simulink model "Funtivities"  (R2023b)
settings: Solver=VariableStepAuto  StartTime=0.0  StopTime=6  RelTol=1e-3
model workspace: external: MATLAB File D:\College\Senior 2\GP\Delta\Design\INSHALLAAHHHHH\SSCPE\Funtivities_DataFile3.m (data not in the file)
undefined symbols (not defined in the file or in its folder): smiData, X, Y, Z
libraries: sm_lib x231, nesl_utility x4
(part 5 of 5)

== system Funtivities/Delta Robot Model/Ta7t_1_RIGID/RodPlusTwoSpheres_2_RIGID ==
  ROd_1_RIGID : Subsystem
  ReferenceFrame : sm_lib/Frames and Transforms/Reference Frame
  Sphere_1_RIGID : Subsystem
  Sphere_2_RIGID : Subsystem
  Transform : sm_lib/Frames and Transforms/Rigid Transform  TranslationMethod=Cartesian  TranslationStandardOffset=0  TranslationStandardOffsetUnits=m  TranslationStandardAxis=+Z  TranslationCartesianOffset=smiData.RigidTransform(59).translation  TranslationCartesianOffsetUnits=mm  TranslationROffset=0  TranslationROffsetUnits=m  TranslationZOffset=0  TranslationZOffsetUnits=m  TranslationThetaOffset=0  TranslationThetaOffsetUnits=deg  RotationMethod=ArbitraryAxis  RotationAngleUnits=rad  RotationStandardAxis=+Z  RotationAngle=smiData.RigidTransform(59).angle  RotationArbitraryAxis=smiData.RigidTransform(59).axis  FollAlignAxisA=+X  BaseAlignAxisA=+Y  FollAlignAxisB=+Y  BaseAlignAxisB=+Z  RotationSequenceAxes=FollowerAxes  RotationSequence=XYX  RotationSequenceAngles=[0 0 0]  RotationSequenceAnglesUnits=deg  RotationMatrix=[1 0 0; 0 1 0; 0 0 1]  Quaternion=[1 0 0 0]
  Transform1 : sm_lib/Frames and Transforms/Rigid Transform  TranslationMethod=Cartesian  TranslationStandardOffset=0  TranslationStandardOffsetUnits=m  TranslationStandardAxis=+Z  TranslationCartesianOffset=smiData.RigidTransform(60).translation  TranslationCartesianOffsetUnits=mm  TranslationROffset=0  TranslationROffsetUnits=m  TranslationZOffset=0  TranslationZOffsetUnits=m  TranslationThetaOffset=0  TranslationThetaOffsetUnits=deg  RotationMethod=ArbitraryAxis  RotationAngleUnits=rad  RotationStandardAxis=+Z  RotationAngle=smiData.RigidTransform(60).angle  RotationArbitraryAxis=smiData.RigidTransform(60).axis  FollAlignAxisA=+X  BaseAlignAxisA=+Y  FollAlignAxisB=+Y  BaseAlignAxisB=+Z  RotationSequenceAxes=FollowerAxes  RotationSequence=XYX  RotationSequenceAngles=[0 0 0]  RotationSequenceAnglesUnits=deg  RotationMatrix=[1 0 0; 0 1 0; 0 0 1]  Quaternion=[1 0 0 0]
  Transform2 : sm_lib/Frames and Transforms/Rigid Transform  TranslationMethod=Cartesian  TranslationStandardOffset=0  TranslationStandardOffsetUnits=m  TranslationStandardAxis=+Z  TranslationCartesianOffset=smiData.RigidTransform(61).translation  TranslationCartesianOffsetUnits=mm  TranslationROffset=0  TranslationROffsetUnits=m  TranslationZOffset=0  TranslationZOffsetUnits=m  TranslationThetaOffset=0  TranslationThetaOffsetUnits=deg  RotationMethod=ArbitraryAxis  RotationAngleUnits=rad  RotationStandardAxis=+Z  RotationAngle=smiData.RigidTransform(61).angle  RotationArbitraryAxis=smiData.RigidTransform(61).axis  FollAlignAxisA=+X  BaseAlignAxisA=+Y  FollAlignAxisB=+Y  BaseAlignAxisB=+Z  RotationSequenceAxes=FollowerAxes  RotationSequence=XYX  RotationSequenceAngles=[0 0 0]  RotationSequenceAnglesUnits=deg  RotationMatrix=[1 0 0; 0 1 0; 0 0 1]  Quaternion=[1 0 0 0]
  Transform3 : sm_lib/Frames and Transforms/Rigid Transform  TranslationMethod=Cartesian  TranslationStandardOffset=0  TranslationStandardOffsetUnits=m  TranslationStandardAxis=+Z  TranslationCartesianOffset=smiData.RigidTransform(62).translation  TranslationCartesianOffsetUnits=mm  TranslationROffset=0  TranslationROffsetUnits=m  TranslationZOffset=0  TranslationZOffsetUnits=m  TranslationThetaOffset=0  TranslationThetaOffsetUnits=deg  RotationMethod=ArbitraryAxis  RotationAngleUnits=rad  RotationStandardAxis=+Z  RotationAngle=smiData.RigidTransform(62).angle  RotationArbitraryAxis=smiData.RigidTransform(62).axis  FollAlignAxisA=+X  BaseAlignAxisA=+Y  FollAlignAxisB=+Y  BaseAlignAxisB=+Z  RotationSequenceAxes=FollowerAxes  RotationSequence=XYX  RotationSequenceAngles=[0 0 0]  RotationSequenceAnglesUnits=deg  RotationMatrix=[1 0 0; 0 1 0; 0 0 1]  Quaternion=[1 0 0 0]
  F : PMIOPort  Side=Right
  connections:
  Sphere_1_RIGID/LConn1 -- Transform/RConn1
  Sphere_2_RIGID/LConn1 -- Transform1/RConn1
  ROd_1_RIGID/LConn1 -- Transform2/RConn1
  Transform/LConn1 -- ReferenceFrame/RConn1 -- Transform1/LConn1 -- Transform2/LConn1 -- Transform3/RConn1
  Transform3/LConn1 -- F/RConn1

== system Funtivities/Delta Robot Model/Ta7t_1_RIGID/RodPlusTwoSpheres_3_RIGID ==
  ROd_1_RIGID : Subsystem
  ReferenceFrame : sm_lib/Frames and Transforms/Reference Frame
  Sphere_1_RIGID : Subsystem
  Sphere_2_RIGID : Subsystem
  Transform : sm_lib/Frames and Transforms/Rigid Transform  TranslationMethod=Cartesian  TranslationStandardOffset=0  TranslationStandardOffsetUnits=m  TranslationStandardAxis=+Z  TranslationCartesianOffset=smiData.RigidTransform(63).translation  TranslationCartesianOffsetUnits=mm  TranslationROffset=0  TranslationROffsetUnits=m  TranslationZOffset=0  TranslationZOffsetUnits=m  TranslationThetaOffset=0  TranslationThetaOffsetUnits=deg  RotationMethod=ArbitraryAxis  RotationAngleUnits=rad  RotationStandardAxis=+Z  RotationAngle=smiData.RigidTransform(63).angle  RotationArbitraryAxis=smiData.RigidTransform(63).axis  FollAlignAxisA=+X  BaseAlignAxisA=+Y  FollAlignAxisB=+Y  BaseAlignAxisB=+Z  RotationSequenceAxes=FollowerAxes  RotationSequence=XYX  RotationSequenceAngles=[0 0 0]  RotationSequenceAnglesUnits=deg  RotationMatrix=[1 0 0; 0 1 0; 0 0 1]  Quaternion=[1 0 0 0]
  Transform1 : sm_lib/Frames and Transforms/Rigid Transform  TranslationMethod=Cartesian  TranslationStandardOffset=0  TranslationStandardOffsetUnits=m  TranslationStandardAxis=+Z  TranslationCartesianOffset=smiData.RigidTransform(64).translation  TranslationCartesianOffsetUnits=mm  TranslationROffset=0  TranslationROffsetUnits=m  TranslationZOffset=0  TranslationZOffsetUnits=m  TranslationThetaOffset=0  TranslationThetaOffsetUnits=deg  RotationMethod=ArbitraryAxis  RotationAngleUnits=rad  RotationStandardAxis=+Z  RotationAngle=smiData.RigidTransform(64).angle  RotationArbitraryAxis=smiData.RigidTransform(64).axis  FollAlignAxisA=+X  BaseAlignAxisA=+Y  FollAlignAxisB=+Y  BaseAlignAxisB=+Z  RotationSequenceAxes=FollowerAxes  RotationSequence=XYX  RotationSequenceAngles=[0 0 0]  RotationSequenceAnglesUnits=deg  RotationMatrix=[1 0 0; 0 1 0; 0 0 1]  Quaternion=[1 0 0 0]
  Transform2 : sm_lib/Frames and Transforms/Rigid Transform  TranslationMethod=Cartesian  TranslationStandardOffset=0  TranslationStandardOffsetUnits=m  TranslationStandardAxis=+Z  TranslationCartesianOffset=smiData.RigidTransform(65).translation  TranslationCartesianOffsetUnits=mm  TranslationROffset=0  TranslationROffsetUnits=m  TranslationZOffset=0  TranslationZOffsetUnits=m  TranslationThetaOffset=0  TranslationThetaOffsetUnits=deg  RotationMethod=ArbitraryAxis  RotationAngleUnits=rad  RotationStandardAxis=+Z  RotationAngle=smiData.RigidTransform(65).angle  RotationArbitraryAxis=smiData.RigidTransform(65).axis  FollAlignAxisA=+X  BaseAlignAxisA=+Y  FollAlignAxisB=+Y  BaseAlignAxisB=+Z  RotationSequenceAxes=FollowerAxes  RotationSequence=XYX  RotationSequenceAngles=[0 0 0]  RotationSequenceAnglesUnits=deg  RotationMatrix=[1 0 0; 0 1 0; 0 0 1]  Quaternion=[1 0 0 0]
  Transform3 : sm_lib/Frames and Transforms/Rigid Transform  TranslationMethod=Cartesian  TranslationStandardOffset=0  TranslationStandardOffsetUnits=m  TranslationStandardAxis=+Z  TranslationCartesianOffset=smiData.RigidTransform(66).translation  TranslationCartesianOffsetUnits=mm  TranslationROffset=0  TranslationROffsetUnits=m  TranslationZOffset=0  TranslationZOffsetUnits=m  TranslationThetaOffset=0  TranslationThetaOffsetUnits=deg  RotationMethod=ArbitraryAxis  RotationAngleUnits=rad  RotationStandardAxis=+Z  RotationAngle=smiData.RigidTransform(66).angle  RotationArbitraryAxis=smiData.RigidTransform(66).axis  FollAlignAxisA=+X  BaseAlignAxisA=+Y  FollAlignAxisB=+Y  BaseAlignAxisB=+Z  RotationSequenceAxes=FollowerAxes  RotationSequence=XYX  RotationSequenceAngles=[0 0 0]  RotationSequenceAnglesUnits=deg  RotationMatrix=[1 0 0; 0 1 0; 0 0 1]  Quaternion=[1 0 0 0]
  F : PMIOPort  Side=Right
  connections:
  Sphere_1_RIGID/LConn1 -- Transform/RConn1
  Sphere_2_RIGID/LConn1 -- Transform1/RConn1
  ROd_1_RIGID/LConn1 -- Transform2/RConn1
  Transform/LConn1 -- ReferenceFrame/RConn1 -- Transform1/LConn1 -- Transform2/LConn1 -- Transform3/RConn1
  Transform3/LConn1 -- F/RConn1

== system Funtivities/Delta Robot Model/Ta7t_1_RIGID/playe_1_RIGID ==
  ReferenceFrame : sm_lib/Frames and Transforms/Reference Frame
  Solid : sm_lib/Body Elements/File Solid  ExtGeomFileName=playe_Default_sldprt.STEP  UnitType=FromFile  ExtGeomFileUnits=m  StepReaderType=HEX  ExportConvexHullGeometry=off  InertiaType=Custom  Mass=smiData.Solid(9).mass  MassUnits=kg  CenterOfMass=smiData.Solid(9).CoM  CenterOfMassUnits=mm  MomentsOfInertia=smiData.Solid(9).MoI  MomentsOfInertiaUnits=kg*mm^2  ProductsOfInertia=smiData.Solid(9).PoI  ProductsOfInertiaUnits=kg*mm^2  BasedOnType=DensityFromFile  Density=1000  DensityUnits=kg/m^3  DoExposeReferenceFrame=on  SerializedFrames=<Frames/>  GraphicType=FromGeometry  MarkerShape=Sphere  MarkerSize=10  GraphicVisPropType=SimpleVisualProperties  GraphicDiffuseColor=smiData.Solid(9).color  GraphicSpecularColor=[0.5 0.5 0.5 1.0]  GraphicAmbientColor=[0.15 0.15 0.15 1.0]  GraphicEmissiveColor=[0.0 0.0 0.0 1.0]  GraphicShininess=75  GraphicOpacity=smiData.Solid(9).opacity
  F : PMIOPort  Side=Left
  connections:
  Solid/RConn1 -- ReferenceFrame/RConn1 -- F/RConn1

== system Funtivities/Delta Robot Model/Ta7t_1_RIGID/RodPlusTwoSpheres_1_RIGID/ROd_1_RIGID ==
  ReferenceFrame : sm_lib/Frames and Transforms/Reference Frame
  Solid : sm_lib/Body Elements/File Solid  ExtGeomFileName=ROd_Default_sldprt.STEP  UnitType=FromFile  ExtGeomFileUnits=m  StepReaderType=HEX  ExportConvexHullGeometry=off  InertiaType=Custom  Mass=smiData.Solid(8).mass  MassUnits=kg  CenterOfMass=smiData.Solid(8).CoM  CenterOfMassUnits=mm  MomentsOfInertia=smiData.Solid(8).MoI  MomentsOfInertiaUnits=kg*mm^2  ProductsOfInertia=smiData.Solid(8).PoI  ProductsOfInertiaUnits=kg*mm^2  BasedOnType=DensityFromFile  Density=1000  DensityUnits=kg/m^3  DoExposeReferenceFrame=on  SerializedFrames=<Frames/>  GraphicType=FromGeometry  MarkerShape=Sphere  MarkerSize=10  GraphicVisPropType=SimpleVisualProperties  GraphicDiffuseColor=smiData.Solid(8).color  GraphicSpecularColor=[0.5 0.5 0.5 1.0]  GraphicAmbientColor=[0.15 0.15 0.15 1.0]  GraphicEmissiveColor=[0.0 0.0 0.0 1.0]  GraphicShininess=75  GraphicOpacity=smiData.Solid(8).opacity
  F : PMIOPort  Side=Left
  connections:
  Solid/RConn1 -- ReferenceFrame/RConn1 -- F/RConn1

== system Funtivities/Delta Robot Model/Ta7t_1_RIGID/RodPlusTwoSpheres_1_RIGID/Sphere_1_RIGID ==
  ReferenceFrame : sm_lib/Frames and Transforms/Reference Frame
  Solid : sm_lib/Body Elements/File Solid  ExtGeomFileName=Sphere_145910-DEBearings_sldprt.STEP  UnitType=FromFile  ExtGeomFileUnits=m  StepReaderType=HEX  ExportConvexHullGeometry=off  InertiaType=Custom  Mass=smiData.Solid(7).mass  MassUnits=kg  CenterOfMass=smiData.Solid(7).CoM  CenterOfMassUnits=mm  MomentsOfInertia=smiData.Solid(7).MoI  MomentsOfInertiaUnits=kg*mm^2  ProductsOfInertia=smiData.Solid(7).PoI  ProductsOfInertiaUnits=kg*mm^2  BasedOnType=DensityFromFile  Density=1000  DensityUnits=kg/m^3  DoExposeReferenceFrame=on  SerializedFrames=<Frames/>  GraphicType=FromGeometry  MarkerShape=Sphere  MarkerSize=10  GraphicVisPropType=SimpleVisualProperties  GraphicDiffuseColor=smiData.Solid(7).color  GraphicSpecularColor=[0.5 0.5 0.5 1.0]  GraphicAmbientColor=[0.15 0.15 0.15 1.0]  GraphicEmissiveColor=[0.0 0.0 0.0 1.0]  GraphicShininess=75  GraphicOpacity=smiData.Solid(7).opacity
  F : PMIOPort  Side=Left
  connections:
  Solid/RConn1 -- ReferenceFrame/RConn1 -- F/RConn1

== system Funtivities/Delta Robot Model/Ta7t_1_RIGID/RodPlusTwoSpheres_1_RIGID/Sphere_2_RIGID ==
  ReferenceFrame : sm_lib/Frames and Transforms/Reference Frame
  Solid : sm_lib/Body Elements/File Solid  ExtGeomFileName=Sphere_145910-DEBearings_sldprt.STEP  UnitType=FromFile  ExtGeomFileUnits=m  StepReaderType=HEX  ExportConvexHullGeometry=off  InertiaType=Custom  Mass=smiData.Solid(7).mass  MassUnits=kg  CenterOfMass=smiData.Solid(7).CoM  CenterOfMassUnits=mm  MomentsOfInertia=smiData.Solid(7).MoI  MomentsOfInertiaUnits=kg*mm^2  ProductsOfInertia=smiData.Solid(7).PoI  ProductsOfInertiaUnits=kg*mm^2  BasedOnType=DensityFromFile  Density=1000  DensityUnits=kg/m^3  DoExposeReferenceFrame=on  SerializedFrames=<Frames/>  GraphicType=FromGeometry  MarkerShape=Sphere  MarkerSize=10  GraphicVisPropType=SimpleVisualProperties  GraphicDiffuseColor=smiData.Solid(7).color  GraphicSpecularColor=[0.5 0.5 0.5 1.0]  GraphicAmbientColor=[0.15 0.15 0.15 1.0]  GraphicEmissiveColor=[0.0 0.0 0.0 1.0]  GraphicShininess=75  GraphicOpacity=smiData.Solid(7).opacity
  F : PMIOPort  Side=Left
  connections:
  Solid/RConn1 -- ReferenceFrame/RConn1 -- F/RConn1

== system Funtivities/Delta Robot Model/Ta7t_1_RIGID/RodPlusTwoSpheres_2_RIGID/ROd_1_RIGID ==
  ReferenceFrame : sm_lib/Frames and Transforms/Reference Frame
  Solid : sm_lib/Body Elements/File Solid  ExtGeomFileName=ROd_Default_sldprt.STEP  UnitType=FromFile  ExtGeomFileUnits=m  StepReaderType=HEX  ExportConvexHullGeometry=off  InertiaType=Custom  Mass=smiData.Solid(8).mass  MassUnits=kg  CenterOfMass=smiData.Solid(8).CoM  CenterOfMassUnits=mm  MomentsOfInertia=smiData.Solid(8).MoI  MomentsOfInertiaUnits=kg*mm^2  ProductsOfInertia=smiData.Solid(8).PoI  ProductsOfInertiaUnits=kg*mm^2  BasedOnType=DensityFromFile  Density=1000  DensityUnits=kg/m^3  DoExposeReferenceFrame=on  SerializedFrames=<Frames/>  GraphicType=FromGeometry  MarkerShape=Sphere  MarkerSize=10  GraphicVisPropType=SimpleVisualProperties  GraphicDiffuseColor=smiData.Solid(8).color  GraphicSpecularColor=[0.5 0.5 0.5 1.0]  GraphicAmbientColor=[0.15 0.15 0.15 1.0]  GraphicEmissiveColor=[0.0 0.0 0.0 1.0]  GraphicShininess=75  GraphicOpacity=smiData.Solid(8).opacity
  F : PMIOPort  Side=Left
  connections:
  Solid/RConn1 -- ReferenceFrame/RConn1 -- F/RConn1

== system Funtivities/Delta Robot Model/Ta7t_1_RIGID/RodPlusTwoSpheres_2_RIGID/Sphere_1_RIGID ==
  ReferenceFrame : sm_lib/Frames and Transforms/Reference Frame
  Solid : sm_lib/Body Elements/File Solid  ExtGeomFileName=Sphere_145910-DEBearings_sldprt.STEP  UnitType=FromFile  ExtGeomFileUnits=m  StepReaderType=HEX  ExportConvexHullGeometry=off  InertiaType=Custom  Mass=smiData.Solid(7).mass  MassUnits=kg  CenterOfMass=smiData.Solid(7).CoM  CenterOfMassUnits=mm  MomentsOfInertia=smiData.Solid(7).MoI  MomentsOfInertiaUnits=kg*mm^2  ProductsOfInertia=smiData.Solid(7).PoI  ProductsOfInertiaUnits=kg*mm^2  BasedOnType=DensityFromFile  Density=1000  DensityUnits=kg/m^3  DoExposeReferenceFrame=on  SerializedFrames=<Frames/>  GraphicType=FromGeometry  MarkerShape=Sphere  MarkerSize=10  GraphicVisPropType=SimpleVisualProperties  GraphicDiffuseColor=smiData.Solid(7).color  GraphicSpecularColor=[0.5 0.5 0.5 1.0]  GraphicAmbientColor=[0.15 0.15 0.15 1.0]  GraphicEmissiveColor=[0.0 0.0 0.0 1.0]  GraphicShininess=75  GraphicOpacity=smiData.Solid(7).opacity
  F : PMIOPort  Side=Left
  connections:
  Solid/RConn1 -- ReferenceFrame/RConn1 -- F/RConn1

== system Funtivities/Delta Robot Model/Ta7t_1_RIGID/RodPlusTwoSpheres_2_RIGID/Sphere_2_RIGID ==
  ReferenceFrame : sm_lib/Frames and Transforms/Reference Frame
  Solid : sm_lib/Body Elements/File Solid  ExtGeomFileName=Sphere_145910-DEBearings_sldprt.STEP  UnitType=FromFile  ExtGeomFileUnits=m  StepReaderType=HEX  ExportConvexHullGeometry=off  InertiaType=Custom  Mass=smiData.Solid(7).mass  MassUnits=kg  CenterOfMass=smiData.Solid(7).CoM  CenterOfMassUnits=mm  MomentsOfInertia=smiData.Solid(7).MoI  MomentsOfInertiaUnits=kg*mm^2  ProductsOfInertia=smiData.Solid(7).PoI  ProductsOfInertiaUnits=kg*mm^2  BasedOnType=DensityFromFile  Density=1000  DensityUnits=kg/m^3  DoExposeReferenceFrame=on  SerializedFrames=<Frames/>  GraphicType=FromGeometry  MarkerShape=Sphere  MarkerSize=10  GraphicVisPropType=SimpleVisualProperties  GraphicDiffuseColor=smiData.Solid(7).color  GraphicSpecularColor=[0.5 0.5 0.5 1.0]  GraphicAmbientColor=[0.15 0.15 0.15 1.0]  GraphicEmissiveColor=[0.0 0.0 0.0 1.0]  GraphicShininess=75  GraphicOpacity=smiData.Solid(7).opacity
  F : PMIOPort  Side=Left
  connections:
  Solid/RConn1 -- ReferenceFrame/RConn1 -- F/RConn1

== system Funtivities/Delta Robot Model/Ta7t_1_RIGID/RodPlusTwoSpheres_3_RIGID/ROd_1_RIGID ==
  ReferenceFrame : sm_lib/Frames and Transforms/Reference Frame
  Solid : sm_lib/Body Elements/File Solid  ExtGeomFileName=ROd_Default_sldprt.STEP  UnitType=FromFile  ExtGeomFileUnits=m  StepReaderType=HEX  ExportConvexHullGeometry=off  InertiaType=Custom  Mass=smiData.Solid(8).mass  MassUnits=kg  CenterOfMass=smiData.Solid(8).CoM  CenterOfMassUnits=mm  MomentsOfInertia=smiData.Solid(8).MoI  MomentsOfInertiaUnits=kg*mm^2  ProductsOfInertia=smiData.Solid(8).PoI  ProductsOfInertiaUnits=kg*mm^2  BasedOnType=DensityFromFile  Density=1000  DensityUnits=kg/m^3  DoExposeReferenceFrame=on  SerializedFrames=<Frames/>  GraphicType=FromGeometry  MarkerShape=Sphere  MarkerSize=10  GraphicVisPropType=SimpleVisualProperties  GraphicDiffuseColor=smiData.Solid(8).color  GraphicSpecularColor=[0.5 0.5 0.5 1.0]  GraphicAmbientColor=[0.15 0.15 0.15 1.0]  GraphicEmissiveColor=[0.0 0.0 0.0 1.0]  GraphicShininess=75  GraphicOpacity=smiData.Solid(8).opacity
  F : PMIOPort  Side=Left
  connections:
  Solid/RConn1 -- ReferenceFrame/RConn1 -- F/RConn1

== system Funtivities/Delta Robot Model/Ta7t_1_RIGID/RodPlusTwoSpheres_3_RIGID/Sphere_1_RIGID ==
  ReferenceFrame : sm_lib/Frames and Transforms/Reference Frame
  Solid : sm_lib/Body Elements/File Solid  ExtGeomFileName=Sphere_145910-DEBearings_sldprt.STEP  UnitType=FromFile  ExtGeomFileUnits=m  StepReaderType=HEX  ExportConvexHullGeometry=off  InertiaType=Custom  Mass=smiData.Solid(7).mass  MassUnits=kg  CenterOfMass=smiData.Solid(7).CoM  CenterOfMassUnits=mm  MomentsOfInertia=smiData.Solid(7).MoI  MomentsOfInertiaUnits=kg*mm^2  ProductsOfInertia=smiData.Solid(7).PoI  ProductsOfInertiaUnits=kg*mm^2  BasedOnType=DensityFromFile  Density=1000  DensityUnits=kg/m^3  DoExposeReferenceFrame=on  SerializedFrames=<Frames/>  GraphicType=FromGeometry  MarkerShape=Sphere  MarkerSize=10  GraphicVisPropType=SimpleVisualProperties  GraphicDiffuseColor=smiData.Solid(7).color  GraphicSpecularColor=[0.5 0.5 0.5 1.0]  GraphicAmbientColor=[0.15 0.15 0.15 1.0]  GraphicEmissiveColor=[0.0 0.0 0.0 1.0]  GraphicShininess=75  GraphicOpacity=smiData.Solid(7).opacity
  F : PMIOPort  Side=Left
  connections:
  Solid/RConn1 -- ReferenceFrame/RConn1 -- F/RConn1

== system Funtivities/Delta Robot Model/Ta7t_1_RIGID/RodPlusTwoSpheres_3_RIGID/Sphere_2_RIGID ==
  ReferenceFrame : sm_lib/Frames and Transforms/Reference Frame
  Solid : sm_lib/Body Elements/File Solid  ExtGeomFileName=Sphere_145910-DEBearings_sldprt.STEP  UnitType=FromFile  ExtGeomFileUnits=m  StepReaderType=HEX  ExportConvexHullGeometry=off  InertiaType=Custom  Mass=smiData.Solid(7).mass  MassUnits=kg  CenterOfMass=smiData.Solid(7).CoM  CenterOfMassUnits=mm  MomentsOfInertia=smiData.Solid(7).MoI  MomentsOfInertiaUnits=kg*mm^2  ProductsOfInertia=smiData.Solid(7).PoI  ProductsOfInertiaUnits=kg*mm^2  BasedOnType=DensityFromFile  Density=1000  DensityUnits=kg/m^3  DoExposeReferenceFrame=on  SerializedFrames=<Frames/>  GraphicType=FromGeometry  MarkerShape=Sphere  MarkerSize=10  GraphicVisPropType=SimpleVisualProperties  GraphicDiffuseColor=smiData.Solid(7).color  GraphicSpecularColor=[0.5 0.5 0.5 1.0]  GraphicAmbientColor=[0.15 0.15 0.15 1.0]  GraphicEmissiveColor=[0.0 0.0 0.0 1.0]  GraphicShininess=75  GraphicOpacity=smiData.Solid(7).opacity
  F : PMIOPort  Side=Left
  connections:
  Solid/RConn1 -- ReferenceFrame/RConn1 -- F/RConn1

== matlab function Funtivities/Inverse Kinematics 1/Inverse kin block Hamz ==
  data: x input; theta1 output; y input; z input; theta2 output; theta3 output
function [theta1,theta2,theta3] = inverse_kin(x,y,z)
%% Entering coords of end-effector 
%x = input("Enter X position of end effector :");
%y = input("Enter Y position of end effector :");
%z = input("Enter Z position of end effector :");
%% calling get-thetas function
%Some delta robot dimensions & constants
SP = 120;    % platform side length
SP = SP*0.5;
SB = 200;    % base  side length
L  = 200;    % driver link length
l  = 360;    % driven link length
delta = 69;  % distance between the each pair of driven links
tau = 100;   % distance between the bearing of the driver link's revolute joint

max_beta = pi/6;   % max angle for the spherical joints
min_angle = -pi/6;  % the minimum angle allowed for the motors
max_angle = pi/3;  % the maximum angle allowed for the motors

wB = (SB*sqrt(3))/(6);
uB = (SB*sqrt(3))/(3);
wP = (SP*sqrt(3))/(6);
uP = (SP*sqrt(3))/(3);

delta_2 = delta/2;
tau_2 = tau/2;

a = wB-uP;
b = (SP-sqrt(3)*wB)/2;
c = wP-0.5*wB;
%constants;
F  = 2*z*L;
% Getting theta 1:
    E_1 = 2*L*(y+a);
    G_1 = x*x + y*y + z*z + a*a + L*L + 2*y*a - l*l;
t_plus1 = (-F + sqrt(((E_1)^2)+((F)^2)-((G_1)^2)))/(G_1-E_1);
t_minus1 = (-F - sqrt(((E_1)^2)+((F)^2)-((G_1)^2)))/(G_1-E_1);
if (abs(t_plus1)>abs(t_minus1))
  t1=t_minus1;
else
  t1=t_plus1;
end
theta1 = 2*atan(t1);
% Getting theta 2:
    E_2 = -L*(sqrt(3)*(x+b)+y+c);
    G_2 = x*x + y*y + z*z + b*b + c*c + L*L + 2*(x*b + y*c) - l*l;
t_plus2 = (-F + sqrt(((E_2)^2)+((F)^2)-((G_2)^2)))/(G_2-E_2);
t_minus2 = (-F - sqrt(((E_2)^2)+((F)^2)-((G_2)^2)))/(G_2-E_2);
if (abs(t_plus2)>abs(t_minus2))
  t2=t_minus2;
else
  t2=t_plus2;
end
theta2 = 2*atan(t2);
% Getting theta 3:
    E_3 = L*(sqrt(3)*(x-b)-y-c);
    G_3 = x*x + y*y + z*z + b*b + c*c + L*L + 2*(-x*b + y*c) - l*l;
t_plus3 = (-F + sqrt(((E_3)^2)+((F)^2)-((G_3)^2)))/(G_3-E_3);
t_minus3 = (-F - sqrt(((E_3)^2)+((F)^2)-((G_3)^2)))/(G_3-E_3);
if (abs(t_plus3)>abs(t_minus3))
  t3=t_minus3;
else
  t3=t_plus3;
end
theta3 = 2*atan(t3);
% saving the three thetas in thetas array

end
%%

== matlab function Funtivities/Inverse Kinematics 1/Inverse kin block1 Hamz  ==
  data: x input; theta1 output; y input; z input; theta2 output; theta3 output
function [theta1,theta2,theta3] = inverse_kin(x,y,z)
%% Entering coords of end-effector 
%x = input("Enter X position of end effector :");
%y = input("Enter Y position of end effector :");
%z = input("Enter Z position of end effector :");
%% calling get-thetas function
%Some delta robot dimensions & constants
SP = 120;    % platform side length
SP = SP*0.5;
SB = 200;    % base  side length
L  = 200;    % driver link length
l  = 360;    % driven link length
delta = 69;  % distance between the each pair of driven links
tau = 100;   % distance between the bearing of the driver link's revolute joint

max_beta = pi/6;   % max angle for the spherical joints
min_angle = -pi/6;  % the minimum angle allowed for the motors
max_angle = pi/3;  % the maximum angle allowed for the motors

wB = (SB*sqrt(3))/(6);
uB = (SB*sqrt(3))/(3);
wP = (SP*sqrt(3))/(6);
uP = (SP*sqrt(3))/(3);

delta_2 = delta/2;
tau_2 = tau/2;

a = wB-uP;
b = (SP-sqrt(3)*wB)/2;
c = wP-0.5*wB;
%constants;
F  = 2*z*L;
% Getting theta 1:
    E_1 = 2*L*(y+a);
    G_1 = x*x + y*y + z*z + a*a + L*L + 2*y*a - l*l;
t_plus1 = (-F + sqrt(((E_1)^2)+((F)^2)-((G_1)^2)))/(G_1-E_1);
t_minus1 = (-F - sqrt(((E_1)^2)+((F)^2)-((G_1)^2)))/(G_1-E_1);
if (abs(t_plus1)>abs(t_minus1))
  t1=t_minus1;
else
  t1=t_plus1;
end
theta1 = 2*atan(t1);
% Getting theta 2:
    E_2 = -L*(sqrt(3)*(x+b)+y+c);
    G_2 = x*x + y*y + z*z + b*b + c*c + L*L + 2*(x*b + y*c) - l*l;
t_plus2 = (-F + sqrt(((E_2)^2)+((F)^2)-((G_2)^2)))/(G_2-E_2);
t_minus2 = (-F - sqrt(((E_2)^2)+((F)^2)-((G_2)^2)))/(G_2-E_2);
if (abs(t_plus2)>abs(t_minus2))
  t2=t_minus2;
else
  t2=t_plus2;
end
theta2 = 2*atan(t2);
% Getting theta 3:
    E_3 = L*(sqrt(3)*(x-b)-y-c);
    G_3 = x*x + y*y + z*z + b*b + c*c + L*L + 2*(-x*b + y*c) - l*l;
t_plus3 = (-F + sqrt(((E_3)^2)+((F)^2)-((G_3)^2)))/(G_3-E_3);
t_minus3 = (-F - sqrt(((E_3)^2)+((F)^2)-((G_3)^2)))/(G_3-E_3);
if (abs(t_plus3)>abs(t_minus3))
  t3=t_minus3;
else
  t3=t_plus3;
end
theta3 = 2*atan(t3);
% saving the three thetas in thetas array

end
%%

== matlab function Funtivities/Trajectory Planning 1/Trajectory block ==
  data: q output; qdot output; q2dot output; t input; qt0 input; qtf input; delta_t input
function [q,qdot,q2dot] = trajectory_planning(t,qt0,qtf,delta_t)
t0=0;
tf=delta_t;
%qt0=-2*pi/6;
%qtf=pi/6;

qt0 = qt0 + pi/2;
qtf = qtf + pi/2;

qdott0=0;
qdottf=0;

A=[1 t0  t0^2 t0^3;0 1 2*t0 3*t0^2;1 tf tf^2 tf^3;0 1 2*tf 3*tf^2];
RHS=[qt0;qdott0;qtf;qdottf];

coeffs=inv(A)*RHS;

%t=linspace(t0,tf,100);
q=coeffs(4)*t.^3+coeffs(3)*t.^2+coeffs(2)*t+coeffs(1);
qdot=3*coeffs(4)*t.^2+2*coeffs(3)*t+coeffs(2);
q2dot=6*coeffs(4)*t+2*coeffs(3);

== matlab function Funtivities/Trajectory Planning 1/Trajectory block1 ==
  data: q output; qdot output; q2dot output; t input; qt0 input; qtf input; delta_t input
function [q,qdot,q2dot] = trajectory_planning(t,qt0,qtf,delta_t)
t0=0;
tf=delta_t;
%qt0=-2*pi/6;
%qtf=pi/6;

qt0 = qt0 + pi/2;
qtf = qtf + pi/2;

qdott0=0;
qdottf=0;


A=[1 t0  t0^2 t0^3;0 1 2*t0 3*t0^2;1 tf tf^2 tf^3;0 1 2*tf 3*tf^2];
RHS=[qt0;qdott0;qtf;qdottf];

coeffs=inv(A)*RHS;

%t=linspace(t0,tf,100);
q=coeffs(4)*t.^3+coeffs(3)*t.^2+coeffs(2)*t+coeffs(1);
qdot=3*coeffs(4)*t.^2+2*coeffs(3)*t+coeffs(2);
q2dot=6*coeffs(4)*t+2*coeffs(3);

== matlab function Funtivities/Trajectory Planning 1/Trajectory block2 ==
  data: q output; qdot output; q2dot output; t input; qt0 input; qtf input; delta_t input
function [q,qdot,q2dot] = trajectory_planning(t,qt0,qtf,delta_t)
t0=0;
tf=delta_t;
%qt0=-2*pi/6;
%qtf=pi/6;

qt0 = qt0 + pi/2;
qtf = qtf + pi/2;

qdott0=0;
qdottf=0;
A=[1 t0  t0^2 t0^3;0 1 2*t0 3*t0^2;1 tf tf^2 tf^3;0 1 2*tf 3*tf^2];
RHS=[qt0;qdott0;qtf;qdottf];

coeffs=inv(A)*RHS;

%t=linspace(t0,tf,100);
q=coeffs(4)*t.^3+coeffs(3)*t.^2+coeffs(2)*t+coeffs(1);
qdot=3*coeffs(4)*t.^2+2*coeffs(3)*t+coeffs(2);
q2dot=6*coeffs(4)*t+2*coeffs(3);
